simulink model "TransitionTypeHandler"  (R2016b)
settings: Solver=FixedStepAuto  StartTime=0.0  StopTime=10.0  RelTol=1e-3  EnableMultiTasking=on
settings Model: Creator=march  LastModifiedBy=snyke7
settings SolverCC: EnableConcurrentExecution=on
settings DataIOCC: SaveFormat=StructureWithTime
settings OptimizationCC: BlockReduction=off  OptimizeBlockIOStorage=off  BufferReuse=off  GlobalBufferReuse=off  ExpressionFolding=off  LocalBlockOutputs=off
settings HardwareCC: ProdBitPerPointer=32  ProdBitPerSizeT=32  ProdBitPerPtrDiffT=32  ProdLargestAtomicFloat=None  ProdWordSize=32  ProdLongLongMode=on  ProdHWDeviceType=Generic->32-bit x86 compatible
settings RTWCC: SystemTargetFile=slrt.tlc  TemplateMakefile=slrt_default_tmf  Description=Simulink Real-Time  RTWCompilerOptimization=on
settings TargetCC: CodeReplacementLibrary=XPC_BLAS  ParMdlRefBuildCompliant=on  ConcurrentExecutionCompliant=on  GeneratePreprocessorConditionals=Use local settings  MatFileLogging=on  MATLABClassNameForMDSCustomization=xpcAperiodicCustomization

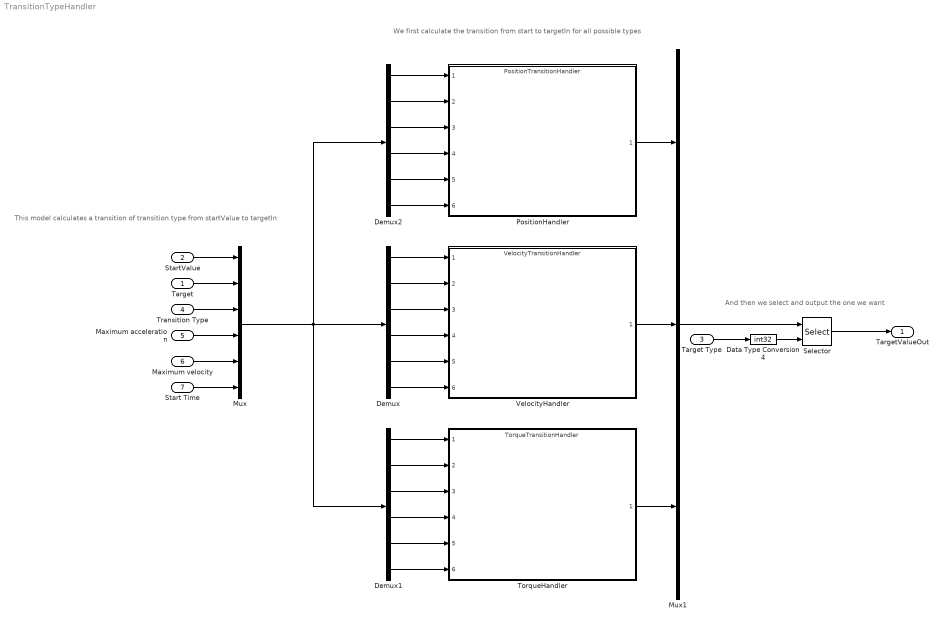
== system TransitionTypeHandler ==
  note: And then we select and output the one we want
  note: We first calculate the transition from start to targetIn for all possible types
  note: This model calculates a transition of transition type from startValue to targetIn
  Target : Inport
  StartValue : Inport  Port=2
  Target Type : Inport  Port=3  OutDataTypeStr=Enum: ControlStrategy
  Transition Type : Inport  Port=4
  Maximum acceleration : Inport  Port=5
  Maximum velocity : Inport  Port=6
  Start Time : Inport  Port=7
  Data Type Conversion4 : DataTypeConversion  OutDataTypeStr=int32
  Demux : Demux  Outputs=6
  Demux1 : Demux  Outputs=6
  Demux2 : Demux  Outputs=6
  Mux : Mux  Inputs=6
  Mux1 : Mux  Inputs=3
  PositionHandler : ModelReference  ModelNameDialog=PositionTransitionHandler  SimulationMode=Normal  ModelReferenceVersion=1.13
  Selector : Selector  InputPortWidth=3  IndexOptions=Index vector (port)  Indices=[1 3]  OutputSizes=1
  TorqueHandler : ModelReference  ModelNameDialog=TorqueTransitionHandler  SimulationMode=Normal  ModelReferenceVersion=1.8
  VelocityHandler : ModelReference  ModelNameDialog=VelocityTransitionHandler  SimulationMode=Normal  ModelReferenceVersion=1.8
  TargetValueOut : Outport
  wires:
  Start Time/1 -> Mux/6
  StartValue/1 -> Mux/1
  Target/1 -> Mux/2
  Maximum acceleration/1 -> Mux/4
  Maximum velocity/1 -> Mux/5
  Demux/1 -> VelocityHandler/1
  Demux/4 -> VelocityHandler/4
  Demux/6 -> VelocityHandler/6
  Demux/5 -> VelocityHandler/5
  Demux/2 -> VelocityHandler/2
  Mux/1 -> Demux/1, Demux1/1, Demux2/1
  Demux1/2 -> TorqueHandler/2
  Demux1/4 -> TorqueHandler/4
  Demux1/5 -> TorqueHandler/5
  Demux1/6 -> TorqueHandler/6
  Demux1/1 -> TorqueHandler/1
  Demux2/1 -> PositionHandler/1
  Demux2/4 -> PositionHandler/4
  Demux2/5 -> PositionHandler/5
  Demux2/2 -> PositionHandler/2
  Demux2/6 -> PositionHandler/6
  VelocityHandler/1 -> Mux1/2
  Mux1/1 -> Selector/1
  Selector/1 -> TargetValueOut/1
  Transition Type/1 -> Mux/3
  Demux1/3 -> TorqueHandler/3
  Demux/3 -> VelocityHandler/3
  Demux2/3 -> PositionHandler/3
  Target Type/1 -> Data Type Conversion4/1
  Data Type Conversion4/1 -> Selector/2
  PositionHandler/1 -> Mux1/1
  TorqueHandler/1 -> Mux1/3
